simulink model "pendulummodel"  (Simulink 7.5)
settings: Solver=ode3  StartTime=0.0  StopTime=100  FixedStep=0.01  RelTol=1e-3
values from neighbouring files (symbols this model uses):
  Dfi_0 = pi/8    (= 0.392699081699)    [simulation.m]
  Dth_0 = 0    [simulation.m]
  fi_0 = 0    [simulation.m]
  th_0 = pi/3    (= 1.0471975512)    [simulation.m]
settings Model: Creator=michal  LastModifiedBy=michal

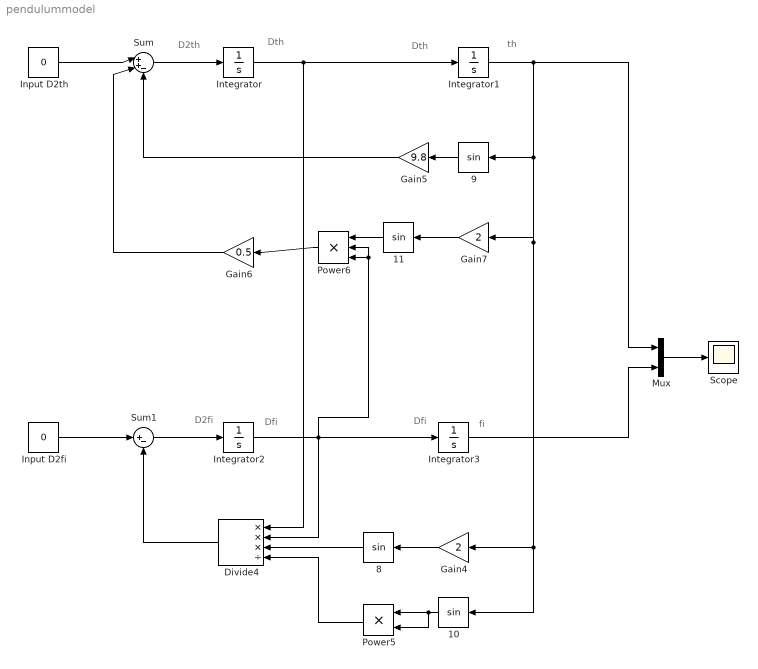
== system pendulummodel ==
  note: D2th
  note: Dth
  note: Dth
  note: th
  note: Dfi
  note: Dfi
  note: fi
  note: D2fi
   {8..11} (4 alike) : Trigonometry
  Divide4 : Product  Inputs=***/  OutDataType=fixdt(1, 16)  OutScaling=2^-10
  Gain4 : Gain  Gain=2  ParameterDataType=fixdt(1, 16)  ParameterScaling=2^0  OutDataType=fixdt(1, 16)  OutScaling=2^0
  Gain5 : Gain  Gain=9.8  ParameterDataType=fixdt(1, 16)  ParameterScaling=2^0  OutDataType=fixdt(1, 16)  OutScaling=2^0
  Gain6 : Gain  Gain=0.5  ParameterDataType=fixdt(1, 16)  ParameterScaling=2^0  OutDataType=fixdt(1, 16)  OutScaling=2^0
  Gain7 : Gain  Gain=2  ParameterDataType=fixdt(1, 16)  ParameterScaling=2^0  OutDataType=fixdt(1, 16)  OutScaling=2^0
  Input D2fi : Constant  Value=0  OutDataType=fixdt(1, 16)  OutScaling=2^0
  Input D2th : Constant  Value=0  OutDataType=fixdt(1, 16)  OutScaling=2^0
  Integrator : Integrator  InitialCondition=Dth_0
  Integrator1 : Integrator  InitialCondition=th_0
  Integrator2 : Integrator  InitialCondition=Dfi_0
  Integrator3 : Integrator  InitialCondition=fi_0
  Mux : Mux  Inputs=2
  Power5 : Product  OutDataType=fixdt(1, 16)  OutScaling=2^0  RndMeth=Zero
  Power6 : Product  Inputs=3  OutDataType=fixdt(1, 16)  OutScaling=2^0  RndMeth=Zero
  Scope : Scope
      settings: YMin=-9000  YMax=12000  SaveName=Angles
  Sum : Sum  Inputs=|++-  OutDataType=fixdt(1, 16)  OutScaling=2^0
  Sum1 : Sum  Inputs=|+-  OutDataType=fixdt(1, 16)  OutScaling=2^0
  wires:
  Integrator/1 -> Integrator1/1, Divide4/1
  Sum/1 -> Integrator/1
  Input D2th/1 -> Sum/1
  Integrator2/1 -> Integrator3/1, Divide4/2, Power6/2, Power6/3
  Integrator1/1 -> Mux/1, " 9"/1, " 10"/1, Gain4/1, Gain7/1
  Integrator3/1 -> Mux/2
  Mux/1 -> Scope/1
  Input D2fi/1 -> Sum1/1
  Sum1/1 -> Integrator2/1
  Gain4/1 -> " 8"/1
  " 8"/1 -> Divide4/3
  " 10"/1 -> Power5/1, Power5/2
  Power5/1 -> Divide4/4
  Divide4/1 -> Sum1/2
  " 9"/1 -> Gain5/1
  Gain5/1 -> Sum/3
  Gain7/1 -> " 11"/1
  " 11"/1 -> Power6/1
  Power6/1 -> Gain6/1
  Gain6/1 -> Sum/2
